simulink model "Sudarshan_question_1"  (R2022b)
settings: Solver=VariableStepAuto  StartTime=0.0  StopTime=1  RelTol=1e-3
libraries: simulink x1, dsparch4 x1
settings Model: Creator=year2  LastModifiedBy=year2

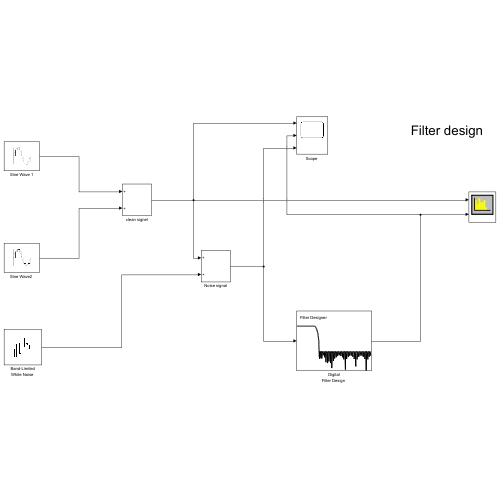
[thumbnail: Simulink's stored preview of the top-level diagram]
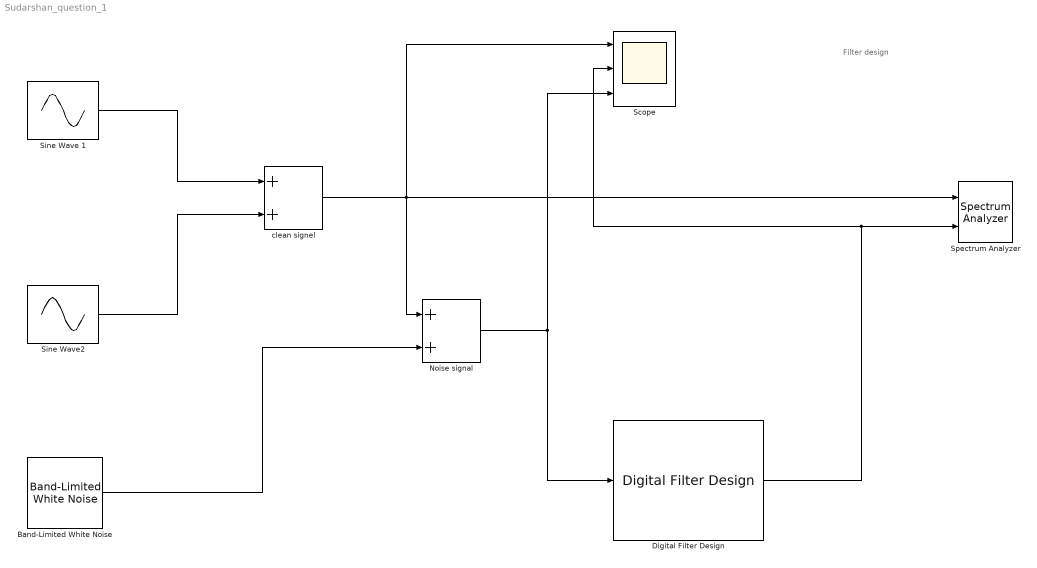
== system Sudarshan_question_1 ==
  note: Filter design
  "Band-Limited White Noise " : simulink/Sources/Band-Limited White Noise  Cov=[0.5]  Ts=0.001  seed=[23341]
  "Digital Filter Design " : dsparch4/Digital Filter Design  mwdsp_browser_bugfix_var=off
  Noise signal : Sum
  "Scope " : Scope  NumInputPorts=3
  Sine Wave 1 : Sin  Frequency=2*pi*50  SampleTime=0.001
  "Sine Wave2 " : Sin  Amplitude=0.5  Frequency=2*pi*200  SampleTime=0.001
  Spectrum Analyzer : SpectrumAnalyzer  NumInputPorts=2
  clean signel : Sum
  wires:
  Sine Wave 1/1 -> clean signel/1
  "Sine Wave2 "/1 -> clean signel/2
  Noise signal/1 -> "Scope "/3, "Digital Filter Design "/1
  "Band-Limited White Noise "/1 -> Noise signal/2
  clean signel/1 -> Noise signal/1, "Scope "/1, Spectrum Analyzer/1
  "Digital Filter Design "/1 -> Spectrum Analyzer/2, "Scope "/2
